simulink model "server_test"  (R2022b)
settings: Solver=VariableStepAuto  StartTime=0.0  StopTime=10.0  RelTol=1e-3
settings Model: Creator=ROG  LastModifiedBy=ROG

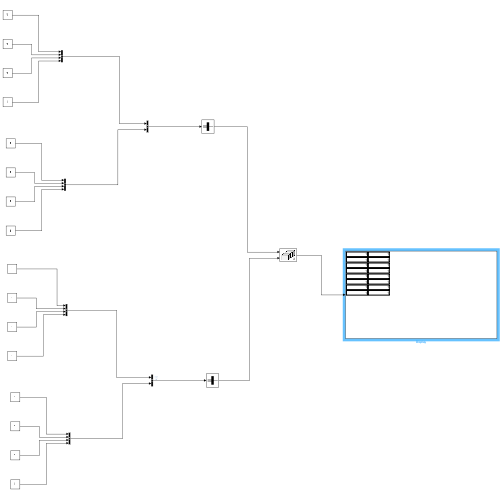
[thumbnail: Simulink's stored preview of the top-level diagram]
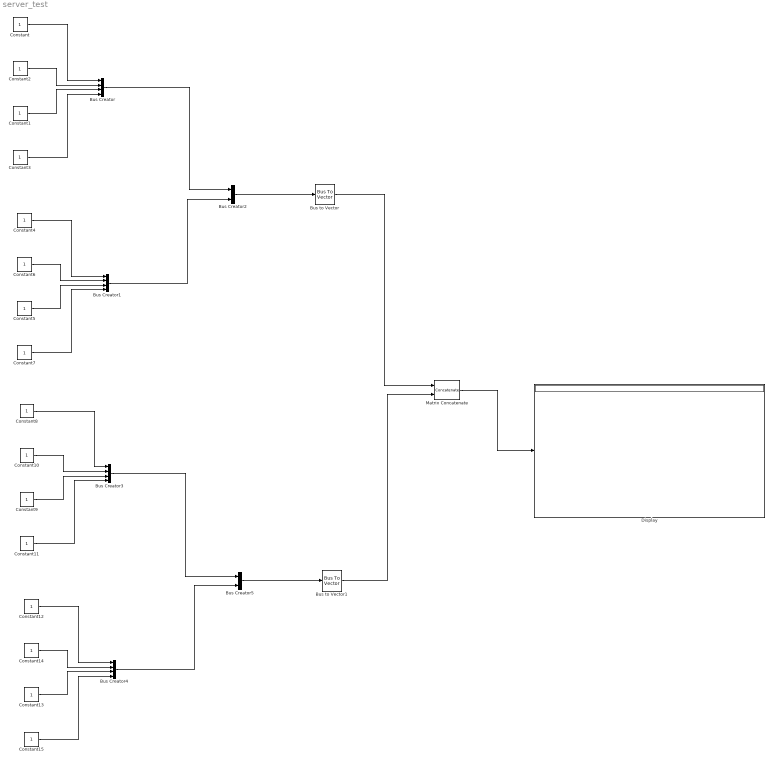
== system server_test ==
  Bus Creator{,1,3..4} (4 alike) : BusCreator  Inputs=4
  Bus Creator2 : BusCreator  Inputs=2
  Bus Creator5 : BusCreator  Inputs=2
  Bus to Vector : BusToVector
  Bus to Vector1 : BusToVector
  Constant{,1..15} (16 alike) : Constant
  Display : Display
  Matrix Concatenate : Concatenate  Mode=Multidimensional array  ConcatenateDimension=2
  wires:
  Constant/1 -> Bus Creator/1
  Constant2/1 -> Bus Creator/2
  Constant1/1 -> Bus Creator/3
  Constant3/1 -> Bus Creator/4
  Bus Creator/1 -> Bus Creator2/1
  Constant7/1 -> Bus Creator1/4
  Constant4/1 -> Bus Creator1/1
  Constant6/1 -> Bus Creator1/2
  Bus Creator1/1 -> Bus Creator2/2
  Constant5/1 -> Bus Creator1/3
  Bus Creator2/1 -> Bus to Vector/1
  Bus Creator5/1 -> Bus to Vector1/1
  Constant9/1 -> Bus Creator3/3
  Constant11/1 -> Bus Creator3/4
  Constant13/1 -> Bus Creator4/3
  Constant14/1 -> Bus Creator4/2
  Bus Creator4/1 -> Bus Creator5/2
  Bus Creator3/1 -> Bus Creator5/1
  Constant8/1 -> Bus Creator3/1
  Constant12/1 -> Bus Creator4/1
  Constant10/1 -> Bus Creator3/2
  Constant15/1 -> Bus Creator4/4
  Bus to Vector/1 -> Matrix Concatenate/1
  Bus to Vector1/1 -> Matrix Concatenate/2
  Matrix Concatenate/1 -> Display/1
